simulink model "OnOffSwitch"  (R2025b)
settings: Solver=VariableStepAuto  StartTime=0.0  StopTime=Inf  RelTol=1e-3
settings Model: Creator=Soochan Kim  LastModifiedBy=Soochan Kim

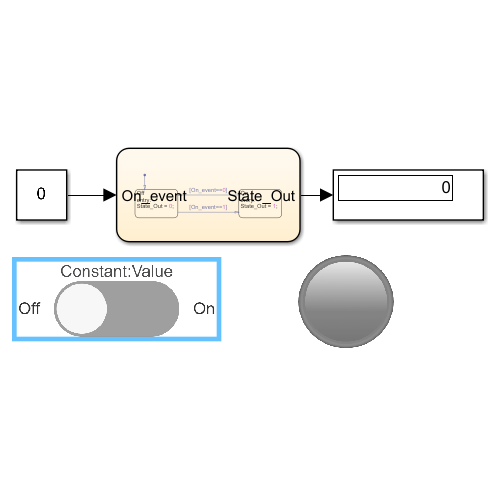
[thumbnail: Simulink's stored preview of the top-level diagram]
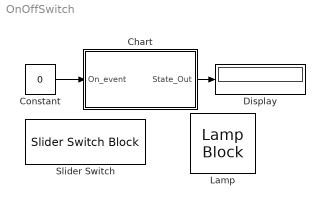
== system OnOffSwitch ==
  Chart : Stateflow chart  TreatAsAtomicUnit=on
  Constant : Constant  Value=0
  Display : Display
  Lamp : LampBlock  LabelPosition=Hide  DefaultColor=[192.0, 192.0, 192.0]
  Slider Switch : SliderSwitchBlock
  wires:
  Chart/1(State_Out) -> Display/1
  Constant/1 -> Chart/1(On_event)

== stateflow chart OnOffSwitch/Chart ==
  settings: updateMethod=DISCRETE  sampleTime=0.1
  state Off
    entry:
    State_Out = 0;
  state On
    entry:
    State_Out = 1;
  (default) -> Off
  On -> Off : [On_event==0]
  Off -> On : [On_event==1]
  data: State_Out output; On_event input
